simulink subsystem "StarCamera"  (R2025b)
settings: Solver=VariableStepAuto  StartTime=0.0  StopTime=10.0  RelTol=1e-3
settings Model: Creator=yvijay  LastModifiedBy=YuktiVijay

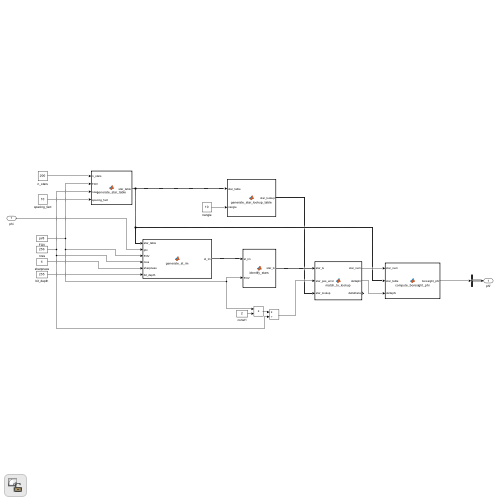
[thumbnail: Simulink's stored preview of the top-level diagram]
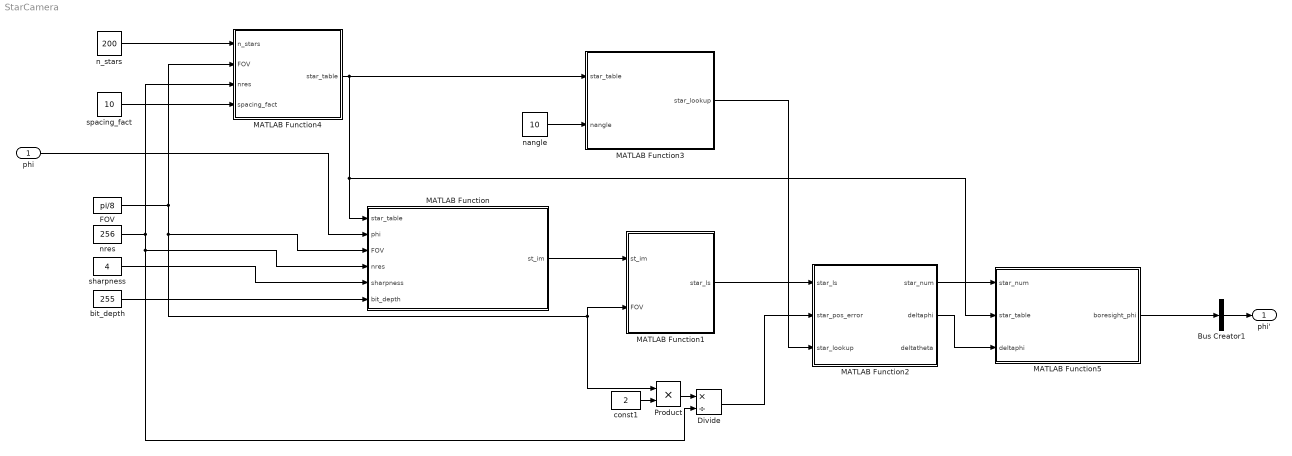
== system StarCamera ==
  phi : Inport
  Bus Creator1 : BusCreator  Inputs=1
  Divide : Product  Inputs=*/
  FOV : Constant  Value=pi/8
  MATLAB Function : MATLAB Function  TreatAsAtomicUnit=on
  MATLAB Function1 : MATLAB Function  TreatAsAtomicUnit=on
  MATLAB Function2 : MATLAB Function  TreatAsAtomicUnit=on
  MATLAB Function3 : MATLAB Function  TreatAsAtomicUnit=on
  MATLAB Function4 : MATLAB Function  TreatAsAtomicUnit=on
  MATLAB Function5 : MATLAB Function  TreatAsAtomicUnit=on
  Product : Product
  bit_depth : Constant  Value=255
  const1 : Constant  Value=2
  n_stars : Constant  Value=200
  nangle : Constant  Value=10
  nres : Constant  Value=256
  sharpness : Constant  Value=4
  spacing_fact : Constant  Value=10
  phi' : Outport
  wires:
  MATLAB Function5/1(boresight_phi) -> Bus Creator1/1
  MATLAB Function2/2(deltaphi) -> MATLAB Function5/3(deltaphi)
  spacing_fact/1 -> MATLAB Function4/4(spacing_fact)
  n_stars/1 -> MATLAB Function4/1(n_stars)
  MATLAB Function4/1(star_table) -> MATLAB Function5/2(star_table), MATLAB Function/1(star_table), MATLAB Function3/1(star_table)
  MATLAB Function3/1(star_lookup) -> MATLAB Function2/3(star_lookup)
  nangle/1 -> MATLAB Function3/2(nangle)
  Divide/1 -> MATLAB Function2/2(star_pos_error)
  Product/1 -> Divide/1
  const1/1 -> Product/2
  MATLAB Function2/1(star_num) -> MATLAB Function5/1(star_num)
  MATLAB Function1/1(star_ls) -> MATLAB Function2/1(star_ls)
  bit_depth/1 -> MATLAB Function/6(bit_depth)
  sharpness/1 -> MATLAB Function/5(sharpness)
  nres/1 -> MATLAB Function4/3(nres), Divide/2, MATLAB Function/4(nres)
  FOV/1 -> Product/1, MATLAB Function1/2(FOV), MATLAB Function/3(FOV), MATLAB Function4/2(FOV)
  MATLAB Function/1(st_im) -> MATLAB Function1/1(st_im)
  phi/1 -> MATLAB Function/2(phi)
  Bus Creator1/1 -> phi'/1

== matlab function StarCamera/MATLAB Function ==
  data: star_table input; st_im output; phi input; FOV input; nres input; sharpness input; bit_depth input
function st_im = generate_st_im(star_table, phi, FOV, nres, sharpness, bit_depth)
    % Input: 
    % star_table: nx3 array, from generate_star_table
    % phi: float, boresight angle of camera, in radians, from -pi to pi
    % FOV: float, angular field of view of camera, in radians, from 0 to 2pi
    % nres: integer, number of pixels on side of image
    % sharpness: float, degree of function describing sun shape (higher
    % is sharper), recommended 1-5
    % bit_depth: integer, max brightness value of each pixel
    % Output: 
    % st_im: nres x nres array, representing synethic star tracker image
    
    % Initialize the output image
    st_im = zeros(nres, nres);

    % Initialize coordinate arrays
    [phi_im,theta_im] = meshgrid(linspace(phi-FOV/2,phi+FOV/2,nres),linspace(-FOV/2,FOV/2,nres));

    % Loop through each star in the star table
    for i = 1:size(star_table, 1)
        iphi = star_table(i, 1); % Azimuth angle
        itheta = star_table(i, 2); % Inclination angle
        ibrightness = star_table(i, 3); % Relative brightness

        if iphi > phi-FOV/2 && iphi < phi+FOV/2 && itheta>-FOV/2 && itheta<FOV/2
            st_im = st_im + ibrightness * bit_depth * exp(-((((phi_im-iphi).^2+(theta_im-itheta).^2)/(10*FOV*ibrightness/nres)^2).^sharpness));
        end
    end

    
    % Add random noise to the image
    noise_level = bit_depth*0.02; % Adjust the noise level as needed
    noise = noise_level * randn(size(st_im)); % Generate Gaussian noise
    st_im = st_im + noise; % Add noise to the image
    st_im(st_im < 0) = 0; % Ensure no negative values

    % Normalize the image to the range [0, 1]
    st_im(st_im>bit_depth) = bit_depth;

    % Invert vertically, not sure why this is needed
    st_im = flipud(st_im);
end

== matlab function StarCamera/MATLAB Function3 ==
  data: star_table input; star_lookup output; nangle input
function star_lookup = generate_star_lookup_table(star_table, nangle)
    % Input
    % star_table: nx3 array, from generate_star_table
    % nangle: integer, how many stars to compute angles to from reference
    % star

    % Output
    % star_lookup: nxnagle array, each row corresponds to given row in
    % star_table, columns are angular distances to nangle closest stars

    % Initialize lookup table
    star_lookup = zeros(size(star_table, 1), nangle);

    % Iterate through each star in the table
    for istar = 1:length(star_table)
        
        % Compute the angular distances from the current star to all other stars
        phi_diff = star_table(istar, 1) - star_table(:, 1);
        theta_diff = star_table(istar, 2) - star_table(:, 2);
        angle_diff = sqrt(phi_diff.^2 + theta_diff.^2);

        % Sort the angular distances and get the indices of the smallest values
        [sorted_angles, ~] = sort(angle_diff);
        star_lookup(istar, :) = sorted_angles(2:min(nangle+1, length(sorted_angles))); % Store the smallest values
    end
end

== matlab function StarCamera/MATLAB Function4 ==
  data: n_stars input; star_table output [..200]; FOV input; nres input; spacing_fact input
function star_table = generate_star_table(n_stars,FOV,nres,spacing_fact)
    % Input: 
    % n_stars: integer, number of stars to include in table
    % FOV: float, angular field of view of camera, in radians, from 0 to 2pi
    % nres: integer, number of pixels on side of image
    % spacing_fact: integer, minimum spacing of stars (as a factor of
    % FOV/nres)

    % Output:
    % star_table: n_stars x 3 array, where column 1 is phi position of
    % star, column 2 is theta position, column 3 is relative brightness
    % (capped at 1)

    % CHANGED FOR CODEGEN n_stars is scalar
    n_stars = n_stars(1);
    % Initialize variables
    iphi = 0;
    itheta = 0;
    ibrightness = 0;

    % Declare empty array
    star_table = zeros(n_stars, 3);

    % Iterate through array, generating random location and brightness
    for istar = 1:n_stars

        % Make sure stars are a set distance apart
        min_dist = spacing_fact*FOV/nres;
        too_close = true;
        if istar > 1
            while too_close
                iphi = -pi/4 + (pi)*rand;
                itheta = -pi/12 + (pi/6)*rand;
                distances = sqrt((iphi-star_table(1:istar,1)).^2+(itheta-star_table(1:istar,2)).^2);
                if min(distances) > min_dist
                    too_close = false;
                end
            end
        else
            iphi = -pi/4 + (pi)*rand;
            itheta = -pi/12 + (pi/6)*rand;
        end
        % Declare parameters for star brightness variation
        mu = 0.5;        % mean
        sigma = 0.1;     % standard deviation
        x_min = 0;    % lower bound
        x_max = 1;     % upper bound
        
        accepted = false;
        while ~accepted
            ibrightness = mu + sigma * randn;
            if ibrightness >= x_min && ibrightness <= x_max
                accepted = true;
            end
        end

        % Save values to present row of array
        star_table(istar,:) = [iphi itheta ibrightness];

    end
end

== matlab function StarCamera/MATLAB Function1 ==
  settings: updateMethod=DISCRETE  sampleTime=0.1
  data: st_im input; star_ls output size=[200 2]; FOV input
function star_ls = identify_stars(st_im, FOV)
 % Input:
% st_im: nxn array, representing image from star tracker
% FOV: float, field of view along each edge of image
% Output:
% star_ls: nx2 array, the phi and theta positions (relative to the
% center of the image) for each star identified

% Get image dimensions (not passed to function call)
 [nres,~] = size(st_im);
% Convert coordinates to phi and theta positions
 phi_positions = linspace(-FOV/2, FOV/2, nres);
 theta_positions = linspace(-FOV/2, FOV/2, nres);
% Identify bright points in the star tracker image
 threshold = 0.5 * max(st_im(:)); % Set a threshold to identify bright points
% Create filtered im
 filtered_im = zeros(size(st_im)); % Initialize filtered image
 filtered_im(st_im > threshold) = 1; % Set values to 1 where st_im exceeds threshold
% Find connected components
 CC = bwconncomp(filtered_im);
% Create label matrix - CHANGED FOR CODEGEN
 L = zeros(size(filtered_im), 'uint16');
 for k = 1:CC.NumObjects
     L(CC.PixelIdxList{k}) = k;
 end
% Create output array for star positions
 star_ls = zeros(max(L(:)), 2);
% Iterate through each connected component
for istar = 1:max(L(:))
% Get the coordinates of the current star cluster
 [y_cluster, x_cluster] = find(L == istar);
% Store the average position of the cluster
 star_ls(istar, 1) = mean(phi_positions(x_cluster)); % Average phi coordinate
 star_ls(istar, 2) = mean(theta_positions(y_cluster)); % Average theta coordinate
end
end

== matlab function StarCamera/MATLAB Function2 ==
  data: star_ls input; star_num output int32 size=1; star_pos_error input; star_lookup input; deltaphi output size=1; deltatheta output size=1
function [star_num,deltaphi,deltatheta] = match_to_lookup(star_ls,star_pos_error,star_lookup)
    % Input
    % star_ls: nx2 array, the phi and theta positions (relative to the
    % center of the image) for each star identified
    % star_pos_error: float, angular uncertainty in position of stars
    % star_lookup: nxnagle array, each row corresponds to given row in
    % star_table, columns are angular distances to closest stars

    % Output
    % star_num: integer, index number of matched star
    % deltaphi: float, offset in phi of matched star from image center, in
    % radians
    % deltatheta: float, offset in phi of matched star from image center,
    % in radians

    % CHANGED FOR CODEGEN Initialize outputs with default values
    star_num = int32(-1);
    deltaphi = 0.0;
    deltatheta = 0.0;

    % Iterate through stars in image, starting closest to middle, until we
    % get a positive match
    star_match = false;
    
    % Calculate the sum of squares for each star position
    star_ls_dist = sum(star_ls.^2, 2);
    
    % Sort the star_ls based on the sum of squares
    [~, sorted_indices] = sort(star_ls_dist);
    star_ls = star_ls(sorted_indices, :);

    istar = 1;
    while star_match == false && istar <= length(star_ls)
        % Compute distances to other stars
        phi_diff = star_ls(istar, 1) - star_ls(:, 1);
        theta_diff = star_ls(istar, 2) - star_ls(:, 2);
        angle_diff = sqrt(phi_diff.^2 + theta_diff.^2);

        % Sort the computed angular distances from smallest to largest
        [sorted_angles, ~] = sort(angle_diff);
        
        % Drop the first element of sorted_angles (distance to itself = 0)
        sorted_angles(1) = [];

        % Reduce sorted angles to only be as long as star_lookup is wide
        sorted_angles = sorted_angles(1:min(length(sorted_angles), size(star_lookup, 2)));

        % Create an array of stars within the positional error range
        match_indices = star_lookup(:, 1) >= (sorted_angles(1) - star_pos_error) & ...
                        star_lookup(:, 1) <= (sorted_angles(1) + star_pos_error);
        matched_stars = star_lookup(match_indices, :);

        % Check if that immediately identified the current state. 
        % If not, compare the angular distances one by one, bringing in more to
        % reduce the number of remaining options
        iangle = 2;

        while size(matched_stars,1) > 1 & iangle <= size(star_lookup,2)
            % fprintf('Found multiple matches, refining to next angle\n')
            
            % We loop through the remaining matches
            for j = 1:size(match_indices, 1)
                if j ~= 0
                    % Check to see if the next closest star is within error of
                    % any of the neighbouring stars listed in the lookup table
                    % If none of the angles are close enough, then reject this
                    % match
                    if all(abs(star_lookup(j, iangle:end) - sorted_angles(iangle)) > star_pos_error)
                        match_indices(j) = 0; % Set the jth non-zero element of match_indices to zero
                    end
                end 
            end
            matched_stars = star_lookup(match_indices, :);
        
            iangle = iangle + 1;
        end
        
        % Check if we could use this star 
        if size(matched_stars,1) ~= 1
            %fprintf('Could not find lookup table match for this star, moving to the next one\n');
            istar = istar + 1; % Move to the next star
        else
            % CHANGED FOR CODEGEN Force scalar by using loop instead of find
            for k = 1:length(match_indices)
                if match_indices(k) ~= 0
                    star_num = int32(k);
                    break;
                end
            end
            deltaphi = star_ls(istar,1); % Offset in phi
            deltatheta = star_ls(istar,2); % Offset in theta
            star_match = true;
            % =fprintf('Matched with star number %d, and it is offset %.4f radians in phi and %.4f radians in theta from boresight\n', star_num, deltaphi, deltatheta);
        end
    end
    
    % Return error if star tracker failed 
    if star_match == false
        % fprintf('Star tracker failed, unable to get a lock on any star.\n')
        star_num = int32(-1);
        deltaphi = 0.0;
        deltatheta = 0.0;
    end
    
end

== matlab function StarCamera/MATLAB Function5 ==
  data: star_num input; boresight_phi output; star_table input; deltaphi input
function boresight_phi = compute_boresight_phi(star_num,star_table,deltaphi)
    % Input
    % star_num: integer, index number of matched star
    % star_table: n_stars x 3 array, where column 1 is phi position of
    % star, column 2 is theta position, column 3 is relative brightness
    % deltaphi: float, offset in phi of matched star from image center, in
    % radians
    
    % Output
    % boresight_phi: float, actual orientation of the center of the cameras
    % FOV [rad]

    boresight_phi = star_table(star_num,1) - deltaphi;
end
